simulink model "verify_DF_fixp16_alu"  (R2020b)
settings: Solver=FixedStepDiscrete  StartTime=0.0  StopTime=0.01  FixedStep=DSPBASampleTime  RelTol=1e-3  EnableMultiTasking=on
PreLoadFcn:
  | setup_verify_DF_fixp16_alu;
InitFcn:
  | setup_verify_DF_fixp16_alu;
values from neighbouring files (symbols this model uses):
  DSPBASampleTime = FoldingFactor / (ClockFrequency * 1e6)    (= 5e-06)    [setup_DF_fixp16_alu_av.m]    (also in setup_sim_DF_fixp16_alu.m; setup_verify_DF_fixp16_alu.m)
undefined symbols (not defined in the file or in its folder): I_max, Position_PI_Limit, sigbuilder_block
libraries: DSPBABase x7, foc_blocks x1
settings Model: Creator=bjeppese  LastModifiedBy=mhonman
settings DataIOCC: LimitDataPoints=on  SaveFormat=Array  ReturnWorkspaceOutputs=off
settings OptimizationCC: LifeSpan=inf
settings DebuggingCC: SolverPrmCheckMsg=warning  SFUnexpectedBacktrackingDiag=warning  SFNoUnconditionalDefaultTransitionDiag=warning  SFExecutionAtInitializationDiag=none  ArithmeticOperatorsInVariantConditions=warning
settings HardwareCC: ProdBitPerPointer=32  ProdBitPerSizeT=32  ProdBitPerPtrDiffT=32  ProdLargestAtomicFloat=None  ProdIntDivRoundTo=Undefined  ProdEndianess=Unspecified  ProdWordSize=32  ProdHWDeviceType=32-bit Generic
settings ModelReferenceCC: PropagateSignalLabelsOutOfModel=off
settings SFSimCC: SimUseLocalCustomCode=off  CustomCodeUndefinedFunction=UseInterfaceOnly
settings RTWCC: RTWUseLocalCustomCode=off
settings CodeAppCC: StateflowObjectComments=on
settings GRTTargetCC: TargetLangStandard=C89/C90 (ANSI)
settings ConfigComp: CovMetricSettings=dw  CovSaveCumulativeToWorkspaceVar=on  CovSaveSingleToWorkspaceVar=on  CovExternalEMLEnable=off

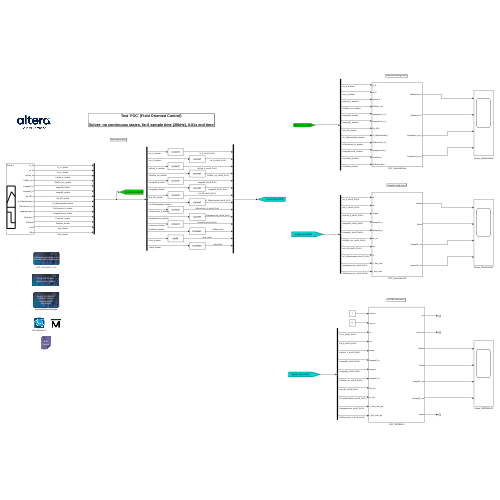
[thumbnail: Simulink's stored preview of the top-level diagram]
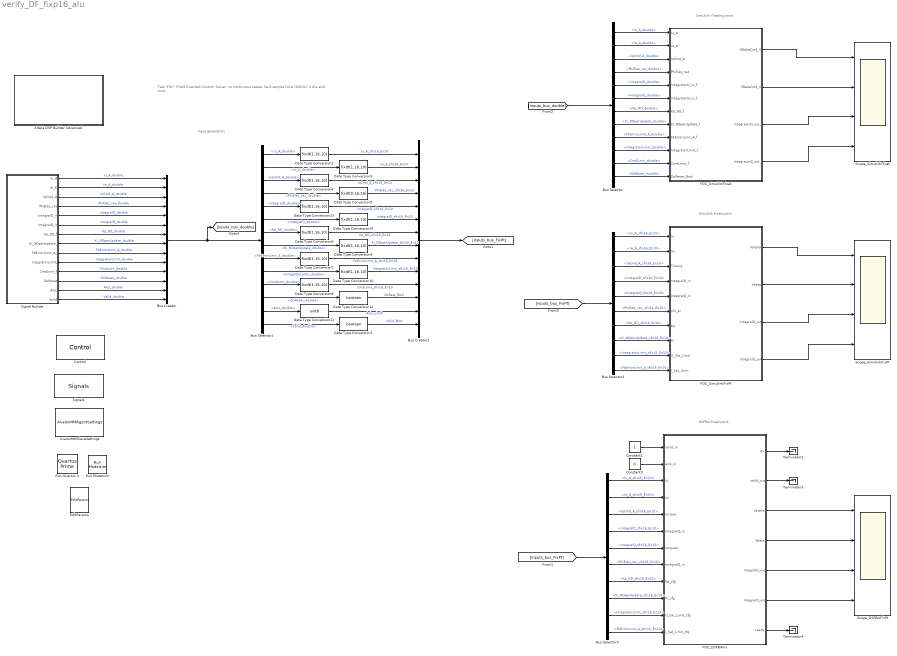
== system verify_DF_fixp16_alu ==
  note: Test 'FOC' (Field Oriented Control)
      |
      | Solver: no continuous states, 5e-6 sample time (20kHz), 0.01s end time
  note: DSPBA fixed point
  note: Input generation
  note: Simulink floating point
  note: Simulink fixed point
  Altera DSP Builder Advanced : Subsystem  mask(DSP Builder Advanced Blockset Ignored Block){}
      settings: OpenFcn=web('http://www.altera.com', '-new');
      mask Display: image(imread('alteralogo.tif'));
  AvalonMMSlaveSettings : DSPBABase/AvalonMMAgentSettings
  Bus Creator : BusCreator  Inputs=14
  Bus Creator1 : BusCreator  Inputs=14
  Bus Selector : BusSelector  OutputSignals=Iu_A_double,Iw_A_double,IqCmd_A_double,PhiElec_rev_double,IntegralD_double,IntegralQ_double,Kp_ND_double,Ki_NDperUpdate_double,FbErrorLimit_A_double,IntegratorLimit_double,CmdLimit_double,DoReset_double
  Bus Selector1 : BusSelector  OutputSignals=Iu_A_double,Iw_A_double,IqCmd_A_double,PhiElec_rev_double,IntegralD_double,IntegralQ_double,Kp_ND_double,Ki_NDperUpdate_double,FbErrorLimit_A_double,IntegratorLimit_double,CmdLimit_double,DoReset_double,Axis_double,Valid_double
  Bus Selector2 : BusSelector  OutputSignals=Iu_A_sfix16_En10,Iw_A_sfix16_En10,IqCmd_A_sfix16_En10,IntegralD_sfix16_En10,IntegralQ_sfix16_En10,PhiElec_rev_ufix16_En16,Kp_ND_sfix16_En10,Ki_NDperUpdate_sfix16_En10,IntegratorLimit_sfix16_En10,FbErrorLimit_A_sfix16_En10
  Bus Selector3 : BusSelector  OutputSignals=Iu_A_sfix16_En10,Iw_A_sfix16_En10,IqCmd_A_sfix16_En10,IntegralD_sfix16_En10,IntegralQ_sfix16_En10,PhiElec_rev_ufix16_En16,Kp_ND_sfix16_En10,Ki_NDperUpdate_sfix16_En10,IntegratorLimit_sfix16_En10,FbErrorLimit_A_sfix16_En10
  Constant1 : Constant  OutDataTypeStr=boolean
  Constant3 : Constant  Value=0  OutDataTypeStr=int32
  Control : DSPBABase/Control  generate=on  language=VHDL  destination=./rtlmax10  destination_gui=./rtlmax10  make_full_path=off  path_is_relative=on  autotestbench=on  signaldepth=2  coveragetestbench=off  logs=off  spacewidth=2  spacenum=1  addrwidth=6  datawidth=32  dataendian=Big Endian  hierarchicalnames=off  ramThresholdBits=-1  distRamThresholdBits=-1  mlabThresholdBits=-1  hardMultiplierThresholdLuts=-1  version=20090407  errorOnChanMismatch=1  errorOnGPIOMismatch=0  importModelsimResults=0  cycleAccurate=off  reinterpretCastMult=off  paramFile=overify_DF_fixp16_alu_params.xml
      settings: AttributesFormatString=HDL Generation is %<generate>
  Data Type Conversion1 : DataTypeConversion  OutDataTypeStr=boolean
  Data Type Conversion{2..4,6..10,13..14} (10 alike) : DataTypeConversion  OutDataTypeStr=fixdt(1,16,10)
  Data Type Conversion11 : DataTypeConversion  OutDataTypeStr=uint8
  Data Type Conversion12 : DataTypeConversion  OutDataTypeStr=boolean
  Data Type Conversion5 : DataTypeConversion  OutDataTypeStr=fixdt(0,16,16)
  EditParams : DSPBABase/EditParams  version=20090407
  FOC_DSPBAFix : Subsystem
  FOC_SimulinkFixPt : Subsystem
  FOC_SimulinkFloat : Subsystem
  Run Modelsim : DSPBABase/Run Modelsim  version=20090407
  Run Quartus II : DSPBABase/Quartus Prime  version=20090407
  Scope_DSPBAFixPt : Scope  NumInputPorts=4
  Scope_SimulinkFixPt : Scope  NumInputPorts=4
  Scope_SimulinkFloat : Scope  NumInputPorts=4
  Signal Builder : Subsystem  Tag=STV Subsys  LoadFcn=sigbuilder_block('load');  StartFcn=sigbuilder_block('start');  StopFcn=sigbuilder_block('stop');  ClipboardFcn=sigbuilder_block('clipboard');  mask(Sigbuilder block){tuvar=[0:10]}
      mask help: Simulink:masks:SigbuilderBlock_MD
      mask init:
      | if ~strcmp(get_param(bdroot(gcbh),'SimulationStatus'),'stopped') tuvar = sigbuilder_block('maskInit'); end
      settings: CopyFcn=sigbuilder_block('copy');  DeleteFcn=sigbuilder_block('delete');  ModelCloseFcn=sigbuilder_block('modelClose');  PreSaveFcn=sigbuilder_block('preSave');  PauseFcn=sigbuilder_block('pause');  ContinueFcn=sigbuilder_block('continue');  NameChangeFcn=sigbuilder_block('namechange');  OpenFcn=sigbuilder_block('open',[6 14.25 1428 732 ]);  CloseFcn=sigbuilder_block('close');
      mask Display: plot(0, 0, 100, 100,[2, 2, 32, 32, 2], [68, 8, 8, 68, 68],[32, 2], [38, 38], [32, 19, 2],[53, 60, 44], [32, 17, 17, 2],[16, 16, 31, 31]);txt = getActiveGroup(gcbh);text(2, 100, txt,'verticalAlignment', 'top');
  Signals : DSPBABase/Signals  clk=clk  freq=ClockFrequency  margin=0  rst=areset  rstactive=High  bus=bus  enbusclock=off  busfreq=100  bussync=on  version=20090407
  Terminator2 : Terminator
  Terminator3 : Terminator
  Terminator4 : Terminator
  wires:
  [inputs_bus_FixPt] -> Bus Selector3/1
  FOC_DSPBAFix/1(qv) -> Terminator2/1
  FOC_DSPBAFix/2(valid_out) -> Terminator3/1
  FOC_DSPBAFix/7(ready) -> Terminator4/1
  FOC_DSPBAFix/3(Valpha) -> Scope_DSPBAFixPt/1
  FOC_DSPBAFix/4(Vbeta) -> Scope_DSPBAFixPt/2
  Constant1/1 -> FOC_DSPBAFix/1(valid_in)
  Constant3/1 -> FOC_DSPBAFix/2(axis_in)
  Bus Selector3/1 -> FOC_DSPBAFix/3(Iu)  "<Iu_A_sfix16_En10>"
  Bus Selector3/2 -> FOC_DSPBAFix/4(Iw)  "<Iw_A_sfix16_En10>"
  Bus Selector3/3 -> FOC_DSPBAFix/5(torque)  "<IqCmd_A_sfix16_En10>"
  Bus Selector3/6 -> FOC_DSPBAFix/8(IntegralD_in)  "<PhiElec_rev_ufix16_En16>"
  Bus Selector3/7 -> FOC_DSPBAFix/9(Kp_cfg)  "<Kp_ND_sfix16_En10>"
  Bus Selector3/8 -> FOC_DSPBAFix/10(Ki_cfg)  "<Ki_NDperUpdate_sfix16_En10>"
  Bus Selector3/9 -> FOC_DSPBAFix/11(U_Sat_Limit_cfg)  "<IntegratorLimit_sfix16_En10>"
  Bus Selector3/10 -> FOC_DSPBAFix/12(I_Sat_Limit_cfg)  "<FbErrorLimit_A_sfix16_En10>"
  Bus Creator/1 -> [inputs_bus_double], Bus Selector1/1
  Bus Creator1/1 -> [inputs_bus_FixPt]
  Signal Builder/9(FbErrorLimit_A_f) -> Bus Creator/9  "FbErrorLimit_A_double"
  Signal Builder/7(Kp_ND_f) -> Bus Creator/7  "Kp_ND_double"
  Signal Builder/8(Ki_NDperUpdate_f) -> Bus Creator/8  "Ki_NDperUpdate_double"
  Signal Builder/10(IntegratorLimit_f) -> Bus Creator/10  "IntegratorLimit_double"
  Signal Builder/11(CmdLimit_f) -> Bus Creator/11  "CmdLimit_double"
  Signal Builder/12(DoReset) -> Bus Creator/12  "DoReset_double"
  Signal Builder/4(PhiElec_rev) -> Bus Creator/4  "PhiElec_rev_double"
  Signal Builder/3(IqCmd_A) -> Bus Creator/3  "IqCmd_A_double"
  Signal Builder/2(Iw_A) -> Bus Creator/2  "Iw_A_double"
  Bus Selector1/1 -> Data Type Conversion2/1  "<Iu_A_double>"
  Data Type Conversion2/1 -> Bus Creator1/1  "Iu_A_sfix16_En10"
  Bus Selector1/2 -> Data Type Conversion3/1  "<Iw_A_double>"
  Data Type Conversion3/1 -> Bus Creator1/2  "Iw_A_sfix16_En10"
  Bus Selector1/3 -> Data Type Conversion4/1  "<IqCmd_A_double>"
  Data Type Conversion4/1 -> Bus Creator1/3  "IqCmd_A_sfix16_En10"
  Bus Selector1/4 -> Data Type Conversion5/1  "<PhiElec_rev_double>"
  Data Type Conversion5/1 -> Bus Creator1/4  "PhiElec_rev_ufix16_En16"
  Bus Selector1/7 -> Data Type Conversion6/1  "<Kp_ND_double>"
  Data Type Conversion6/1 -> Bus Creator1/7  "Kp_ND_sfix16_En10"
  Bus Selector1/8 -> Data Type Conversion9/1  "<Ki_NDperUpdate_double>"
  Data Type Conversion9/1 -> Bus Creator1/8  "Ki_NDperUpdate_sfix16_En10"
  Bus Selector1/9 -> Data Type Conversion7/1  "<FbErrorLimit_A_double>"
  Data Type Conversion7/1 -> Bus Creator1/9  "FbErrorLimit_A_sfix16_En10"
  Bus Selector1/10 -> Data Type Conversion10/1  "<IntegratorLimit_double>"
  Data Type Conversion10/1 -> Bus Creator1/10  "IntegratorLimit_sfix16_En10"
  Bus Selector1/11 -> Data Type Conversion8/1  "<CmdLimit_double>"
  Data Type Conversion8/1 -> Bus Creator1/11  "CmdLimit_sfix16_En10"
  Bus Selector1/12 -> Data Type Conversion12/1  "<DoReset_double>"
  Signal Builder/13(Axis) -> Bus Creator/13  "Axis_double"
  Bus Selector1/13 -> Data Type Conversion11/1  "<Axis_double>"
  Data Type Conversion11/1 -> Bus Creator1/13  "Axis_uint8"
  Signal Builder/14(Valid) -> Bus Creator/14  "Valid_double"
  Data Type Conversion12/1 -> Bus Creator1/12  "DoRest_Bool"
  Bus Selector1/14 -> Data Type Conversion1/1  "<Valid_double>"
  Data Type Conversion1/1 -> Bus Creator1/14  "Valid_Bool"
  Signal Builder/1(Iu_A) -> Bus Creator/1  "Iu_A_double"
  Signal Builder/6(IntegralQ_in) -> Bus Creator/6  "IntegralQ_double"
  Signal Builder/5(IntegralD_in) -> Bus Creator/5  "IntegralD_double"
  Bus Selector1/5 -> Data Type Conversion13/1  "<IntegralD_double>"
  Data Type Conversion13/1 -> Bus Creator1/5  "IntegralD_sfix16_En10"
  Data Type Conversion14/1 -> Bus Creator1/6  "IntegralQ_sfix16_En10"
  Bus Selector1/6 -> Data Type Conversion14/1  "<IntegralQ_double>"
  Bus Selector3/4 -> FOC_DSPBAFix/6(IntegralQ_in)  "<IntegralD_sfix16_En10>"
  Bus Selector3/5 -> FOC_DSPBAFix/7(torque2)  "<IntegralQ_sfix16_En10>"
  FOC_DSPBAFix/5(IntegralD_out) -> Scope_DSPBAFixPt/3
  FOC_DSPBAFix/6(IntegralQ_out) -> Scope_DSPBAFixPt/4
  [inputs_bus_FixPt] -> Bus Selector2/1
  [inputs_bus_double] -> Bus Selector/1
  FOC_SimulinkFixPt/1(Valpha) -> Scope_SimulinkFixPt/1
  FOC_SimulinkFixPt/2(Vbeta) -> Scope_SimulinkFixPt/2
  FOC_SimulinkFloat/1(VAlphaCmd_V) -> Scope_SimulinkFloat/1
  FOC_SimulinkFloat/2(VBetaCmd_V) -> Scope_SimulinkFloat/2
  Bus Selector/1 -> FOC_SimulinkFloat/1(Iu_A)  "<Iu_A_double>"
  Bus Selector/2 -> FOC_SimulinkFloat/2(Iw_A)  "<Iw_A_double>"
  Bus Selector/3 -> FOC_SimulinkFloat/3(IqCmd_A)  "<IqCmd_A_double>"
  Bus Selector/4 -> FOC_SimulinkFloat/4(PhiElec_rad)  "<PhiElec_rev_double>"
  Bus Selector/7 -> FOC_SimulinkFloat/7(Kp_ND_f)  "<Kp_ND_double>"
  Bus Selector/8 -> FOC_SimulinkFloat/8(Ki_NDperUpdate_f)  "<Ki_NDperUpdate_double>"
  Bus Selector/9 -> FOC_SimulinkFloat/9(FbErrorLimit_A_f)  "<FbErrorLimit_A_double>"
  Bus Selector/10 -> FOC_SimulinkFloat/10(IntegratorLimit_f)  "<IntegratorLimit_double>"
  Bus Selector/11 -> FOC_SimulinkFloat/11(CmdLimit_f)  "<CmdLimit_double>"
  Bus Selector/12 -> FOC_SimulinkFloat/12(DoReset_Bool)  "<DoReset_double>"
  Bus Selector2/1 -> FOC_SimulinkFixPt/1(Iu)  "<Iu_A_sfix16_En10>"
  Bus Selector2/2 -> FOC_SimulinkFixPt/2(Iw)  "<Iw_A_sfix16_En10>"
  Bus Selector2/3 -> FOC_SimulinkFixPt/3(Torque)  "<IqCmd_A_sfix16_En10>"
  Bus Selector2/6 -> FOC_SimulinkFixPt/6(phi_el)  "<PhiElec_rev_ufix16_En16>"
  Bus Selector2/7 -> FOC_SimulinkFixPt/7(Kp)  "<Kp_ND_sfix16_En10>"
  Bus Selector2/8 -> FOC_SimulinkFixPt/8(Ki)  "<Ki_NDperUpdate_sfix16_En10>"
  Bus Selector2/9 -> FOC_SimulinkFixPt/9(U_Sat_Limit)  "<IntegratorLimit_sfix16_En10>"
  Bus Selector2/10 -> FOC_SimulinkFixPt/10(I_Sat_Limit)  "<FbErrorLimit_A_sfix16_En10>"
  Bus Selector2/4 -> FOC_SimulinkFixPt/4(IntegralD_in)  "<IntegralD_sfix16_En10>"
  Bus Selector2/5 -> FOC_SimulinkFixPt/5(IntegralQ_in)  "<IntegralQ_sfix16_En10>"
  FOC_SimulinkFixPt/3(IntegralD_out) -> Scope_SimulinkFixPt/3
  FOC_SimulinkFixPt/4(IntegralQ_out) -> Scope_SimulinkFixPt/4
  Bus Selector/5 -> FOC_SimulinkFloat/5(IntegratorD_in_f)  "<IntegralD_double>"
  Bus Selector/6 -> FOC_SimulinkFloat/6(IntegratorQ_in_f)  "<IntegralQ_double>"
  FOC_SimulinkFloat/3(IntegratorD_out_f) -> Scope_SimulinkFloat/3
  FOC_SimulinkFloat/4(IntegratorQ_out_f) -> Scope_SimulinkFloat/4

== system verify_DF_fixp16_alu/Altera DSP Builder Advanced ==

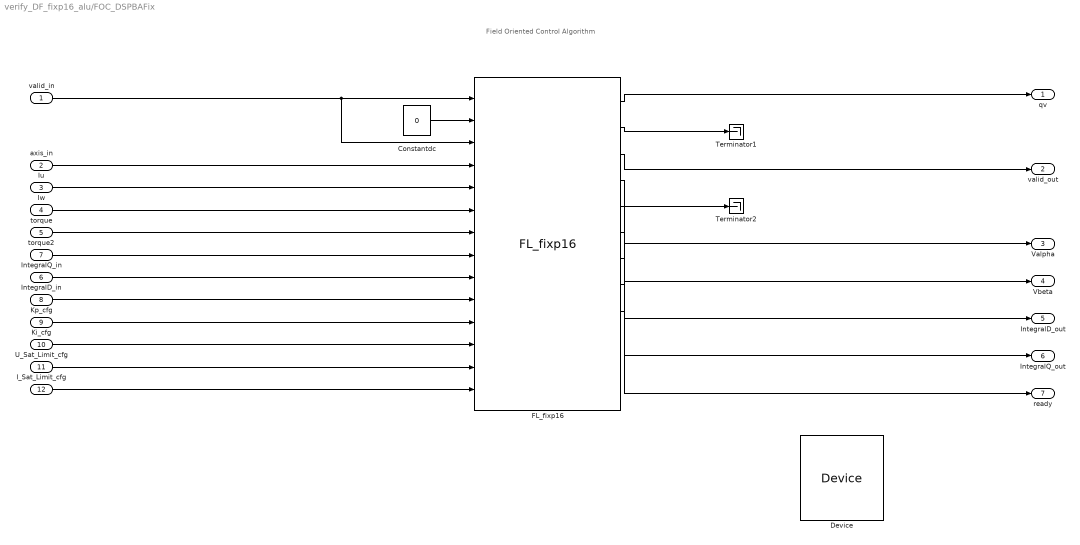
== system verify_DF_fixp16_alu/FOC_DSPBAFix ==
  note: Field Oriented Control Algorithm
  valid_in : Inport
  axis_in : Inport  Port=2
  Iu : Inport  Port=3
  Iw : Inport  Port=4
  torque : Inport  Port=5
  IntegralQ_in : Inport  Port=6
  torque2 : Inport  Port=7
  IntegralD_in : Inport  Port=8
  Kp_cfg : Inport  Port=9
  Ki_cfg : Inport  Port=10
  U_Sat_Limit_cfg : Inport  Port=11
  I_Sat_Limit_cfg : Inport  Port=12
  Constantdc : Constant  Value=0  OutDataTypeStr=uint8  SampleTime=DSPBASampleTime
  Device : DSPBABase/Device  family=MAX 10  deviceMember=Stratix V GX  stratix4device=Stratix IV E  hardcopy4device=HardCopy IV E  stratix5device=Stratix V GX  device=AUTO  speed=6  stratixSpeed=-5  stratix2Speed=-3  stratix3Speed=-2  stratix4gxSpeed=-2  stratix4gtSpeed=-1  cyclone2Speed=-6  cyclone3Speed=-7  arria2Speed=-4  cyclone4eSpeed=-8  stratix5Speed=-3  arria5Speed=-4  arriaSpeed=-6  cyclone3lsSpeed=-7  cyclone5Speed=-6  arria2gzSpeed=-3  nightFurySpeed=-2  ecp2Speed=-7  hardcopycompat=off  version=20140217  max10flashmode=off  max10nomeminit=off
  FL_fixp16 : foc_blocks/FL_fixp16  SystemSampleTime=-1  VariantActivationTime=update diagram  Latency=0  AutoFrameSizeCalculation=off
      link override ChannelOut1: latency=19
      settings: SourceProductName=FOC Blocks
  Terminator1 : Terminator
  Terminator2 : Terminator
  qv : Outport
  valid_out : Outport  Port=2
  Valpha : Outport  Port=3
  Vbeta : Outport  Port=4
  IntegralD_out : Outport  Port=5
  IntegralQ_out : Outport  Port=6
  ready : Outport  Port=7
  wires:
  FL_fixp16/5 -> Valpha/1
  FL_fixp16/1 -> qv/1
  FL_fixp16/3 -> valid_out/1
  FL_fixp16/6 -> Vbeta/1
  Constantdc/1 -> FL_fixp16/2
  FL_fixp16/8 -> IntegralQ_out/1
  FL_fixp16/7 -> IntegralD_out/1
  FL_fixp16/2 -> Terminator1/1
  valid_in/1 -> FL_fixp16/3, FL_fixp16/1
  Iu/1 -> FL_fixp16/5
  Iw/1 -> FL_fixp16/6
  torque/1 -> FL_fixp16/7
  IntegralD_in/1 -> FL_fixp16/10
  Kp_cfg/1 -> FL_fixp16/11
  Ki_cfg/1 -> FL_fixp16/12
  U_Sat_Limit_cfg/1 -> FL_fixp16/13
  axis_in/1 -> FL_fixp16/4
  FL_fixp16/9 -> ready/1
  FL_fixp16/4 -> Terminator2/1
  IntegralQ_in/1 -> FL_fixp16/9
  torque2/1 -> FL_fixp16/8
  I_Sat_Limit_cfg/1 -> FL_fixp16/14

== system verify_DF_fixp16_alu/FOC_SimulinkFixPt ==
  Iu : Inport
  Iw : Inport  Port=2
  Torque : Inport  Port=3
  IntegralD_in : Inport  Port=4
  IntegralQ_in : Inport  Port=5
  phi_el : Inport  Port=6
  Kp : Inport  Port=7
  Ki : Inport  Port=8
  U_Sat_Limit : Inport  Port=9
  I_Sat_Limit : Inport  Port=10
  FL_1 : Subsystem
  Valpha : Outport
  Vbeta : Outport  Port=2
  IntegralD_out : Outport  Port=3
  IntegralQ_out : Outport  Port=4
  wires:
  Iu/1 -> FL_1/1(Iu)
  Iw/1 -> FL_1/2(Iw)
  Torque/1 -> FL_1/3(Torque)
  phi_el/1 -> FL_1/6(phi_el)
  Kp/1 -> FL_1/7(Kp)
  Ki/1 -> FL_1/8(Ki)
  U_Sat_Limit/1 -> FL_1/9(U_Sat_Limit)
  I_Sat_Limit/1 -> FL_1/10(I_Sat_Limit)
  FL_1/1(Valpha) -> Valpha/1
  FL_1/2(Vbeta) -> Vbeta/1
  IntegralD_in/1 -> FL_1/5(IntegralD_in)
  IntegralQ_in/1 -> FL_1/4(IntegralQ_in)
  FL_1/3(IntegralD_out) -> IntegralD_out/1
  FL_1/4(IntegralQ_out) -> IntegralQ_out/1

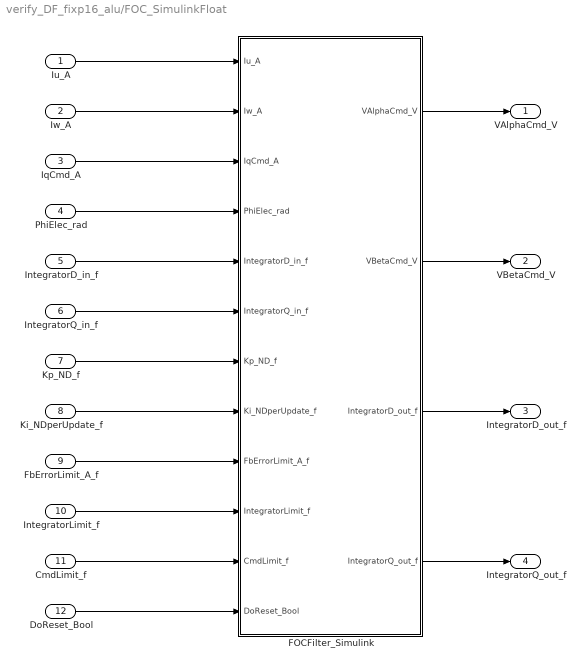
== system verify_DF_fixp16_alu/FOC_SimulinkFloat ==
  Iu_A : Inport
  Iw_A : Inport  Port=2
  IqCmd_A : Inport  Port=3
  PhiElec_rad : Inport  Port=4
  IntegratorD_in_f : Inport  Port=5
  IntegratorQ_in_f : Inport  Port=6
  Kp_ND_f : Inport  Port=7
  Ki_NDperUpdate_f : Inport  Port=8
  FbErrorLimit_A_f : Inport  Port=9
  IntegratorLimit_f : Inport  Port=10
  CmdLimit_f : Inport  Port=11
  DoReset_Bool : Inport  Port=12
  FOCFilter_Simulink : Subsystem
  VAlphaCmd_V : Outport
  VBetaCmd_V : Outport  Port=2
  IntegratorD_out_f : Outport  Port=3
  IntegratorQ_out_f : Outport  Port=4
  wires:
  IqCmd_A/1 -> FOCFilter_Simulink/3(IqCmd_A)
  Iu_A/1 -> FOCFilter_Simulink/1(Iu_A)
  Iw_A/1 -> FOCFilter_Simulink/2(Iw_A)
  PhiElec_rad/1 -> FOCFilter_Simulink/4(PhiElec_rad)
  Kp_ND_f/1 -> FOCFilter_Simulink/7(Kp_ND_f)
  Ki_NDperUpdate_f/1 -> FOCFilter_Simulink/8(Ki_NDperUpdate_f)
  FbErrorLimit_A_f/1 -> FOCFilter_Simulink/9(FbErrorLimit_A_f)
  IntegratorLimit_f/1 -> FOCFilter_Simulink/10(IntegratorLimit_f)
  CmdLimit_f/1 -> FOCFilter_Simulink/11(CmdLimit_f)
  DoReset_Bool/1 -> FOCFilter_Simulink/12(DoReset_Bool)
  FOCFilter_Simulink/1(VAlphaCmd_V) -> VAlphaCmd_V/1
  FOCFilter_Simulink/2(VBetaCmd_V) -> VBetaCmd_V/1
  IntegratorD_in_f/1 -> FOCFilter_Simulink/5(IntegratorD_in_f)
  IntegratorQ_in_f/1 -> FOCFilter_Simulink/6(IntegratorQ_in_f)
  FOCFilter_Simulink/3(IntegratorD_out_f) -> IntegratorD_out_f/1
  FOCFilter_Simulink/4(IntegratorQ_out_f) -> IntegratorQ_out_f/1

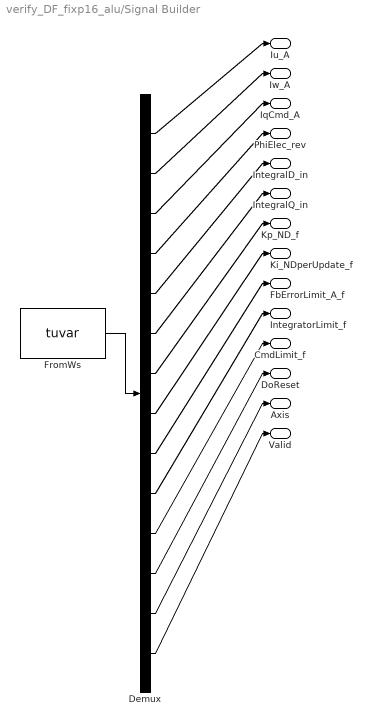
== system verify_DF_fixp16_alu/Signal Builder ==
  Demux : Demux  Tag=STV Demux  Outputs=14
      settings: DisplayOption=none
  FromWs : FromWorkspace  Tag=STV FromWs  VariableName=tuvar  SampleTime=DSPBASampleTime
      SigBuilderData=|
      | common.afterFinalStr = 'Extrapolate'
      | common.sampleTime = 'DSPBASampleTime'
      | dataSet.timeRange = [0 0.01]
      | dataSet.name = 'Group 1'
      | sbobj.Groups.Name = 'Group 1'
      | sbobj.Groups.Signals(1).Name = 'Iu_A'
      | sbobj.Groups.Signals(1).XData = [0 0.0011 0.0011 0.00256 0.00256 0.005 0.005 0.00625 0.00625 0.0075 0.0075 0.00875 0.00875 0.01]
      | sbobj.Groups.Signals(1).YData = [0 0 0.8 0.8 -0.6 -0.6 0.5 0.5 -0.6 -0.6 0.8 0.8 -0.85 -0.85]
      | sbobj.Groups.Signals(2).Name = 'Iw_A'
      | sbobj.Groups.Signals(2).XData = [0 0.00126 0.00126 0.00273 0.00273 0.00483 0.00483 0.00608 0.00608 0.0075 0.0075 0.00875 0.00875 0.01]
      | sbobj.Groups.Signals(2).YData = [0 0 0.7 0.7 -0.6 -0.6 0.6 0.6 -0.7 -0.7 0.6 0.6 -0.85 -0.85]
      | sbobj.Groups.Signals(3).Name = 'IqCmd_A'
      | sbobj.Groups.Signals(3).XData = [0 0.00146 0.00146 0.00292 0.00292 0.00473 0.00473 0.00595 0.00595 0.0075 0.0075 0.00875 0.00875 0.01]
      | sbobj.Groups.Signals(3).YData = [0 0 0.7 0.7 -0.95 -0.95 0.6 0.6 -0.8 -0.8 0.55 0.55 -0.7 -0.7]
      | sbobj.Groups.Signals(4).Name = 'PhiElec_rev'
      | sbobj.Groups.Signals(4).XData = [0 0.00161 0.00161 0.00309 0.00309 0.00462 0.00462 0.00582 0.00582 0.0075 0.0075 0.00875 0.00875 0.01]
      | sbobj.Groups.Signals(4).YData = [0 0 0.9 0.9 -0.95 -0.95 0.65 0.65 -0.95 -0.95 0.9 0.9 -0.65 -0.65]
      | sbobj.Groups.Signals(5).Name = 'IntegralD_in'
      | sbobj.Groups.Signals(5).XData = [0 0.00172 0.00172 0.0033 0.0033 0.00442 0.00442 0.00567 0.00567 0.0075 0.0075 0.00875 0.00875 0.01]
      | sbobj.Groups.Signals(5).YData = [0 0 0.65 0.65 -0.75 -0.75 0.8 0.8 -0.7 -0.7 0.8 0.8 -0.6 -0.6]
      | sbobj.Groups.Signals(6).Name = 'IntegralQ_in'
      | sbobj.Groups.Signals(6).XData = [0 0.00191 0.00191 0.00341 0.00341 0.00422 0.00422 0.00547 0.00547 0.0075 0.0075 0.00875 0.00875 0.01]
      | sbobj.Groups.Signals(6).YData = [0 0 0.8 0.8 -0.7 -0.7 0.8 0.8 -0.6 -0.6 0.7 0.7 -0.65 -0.65]
      | sbobj.Groups.Signals(7).Name = 'Kp_ND_f'
      | sbobj.Groups.Signals(7).XData = [0 0.01]
      | sbobj.Groups.Signals(7).YData = [0.1953125 0.1953125]
      | sbobj.Groups.Signals(8).Name = 'Ki_NDperUpdate_f'
      | sbobj.Groups.Signals(8).XData = [0 0.01]
      | sbobj.Groups.Signals(8).YData = [0.009765625 0.009765625]
      | sbobj.Groups.Signals(9).Name = 'FbErrorLimit_A_f'
      | sbobj.Groups.Signals(9).XData = [0 0.01]
      | sbobj.Groups.Signals(9).YData = [3.051757813 3.051757813]
      | sbobj.Groups.Signals(10).Name = 'IntegratorLimit_f'
      | sbobj.Groups.Signals(10).XData = [0 0.01]
      | sbobj.Groups.Signals(10).YData = [2.9296875 2.9296875]
      | sbobj.Groups.Signals(11).Name = 'CmdLimit_f'
      | sbobj.Groups.Signals(11).XData = [0 0.01]
      | sbobj.Groups.Signals(11).YData = [2.9296875 2.9296875]
      | sbobj.Groups.Signals(12).Name = 'DoReset'
      | sbobj.Groups.Signals(12).XData = [0 0.00047 0.00047 0.01]
      | sbobj.Groups.Signals(12).YData = [1 1 0 0]
      | sbobj.Groups.Signals(13).Name = 'Axis'
      | sbobj.Groups.Signals(13).XData = [0 0.01]
      | sbobj.Groups.Signals(13).YData = [0 0]
      | sbobj.Groups.Signals(14).Name = 'Valid'
      | sbobj.Groups.Signals(14).XData = [0 0.00066 0.00066 0.01]
      | sbobj.Groups.Signals(14).YData = [0 0 1 1]
      | sbobj.Groups.TimeRange = [0 0.01]
  Iu_A : Outport  Tag=STV Outport
  Iw_A : Outport  Tag=STV Outport  Port=2
  IqCmd_A : Outport  Tag=STV Outport  Port=3
  PhiElec_rev : Outport  Tag=STV Outport  Port=4
  IntegralD_in : Outport  Tag=STV Outport  Port=5
  IntegralQ_in : Outport  Tag=STV Outport  Port=6
  Kp_ND_f : Outport  Tag=STV Outport  Port=7
  Ki_NDperUpdate_f : Outport  Tag=STV Outport  Port=8
  FbErrorLimit_A_f : Outport  Tag=STV Outport  Port=9
  IntegratorLimit_f : Outport  Tag=STV Outport  Port=10
  CmdLimit_f : Outport  Tag=STV Outport  Port=11
  DoReset : Outport  Tag=STV Outport  Port=12
  Axis : Outport  Tag=STV Outport  Port=13
  Valid : Outport  Tag=STV Outport  Port=14
  wires:
  FromWs/1 -> Demux/1
  Demux/1 -> Iu_A/1
  Demux/2 -> Iw_A/1
  Demux/3 -> IqCmd_A/1
  Demux/4 -> PhiElec_rev/1
  Demux/5 -> IntegralD_in/1
  Demux/6 -> IntegralQ_in/1
  Demux/7 -> Kp_ND_f/1
  Demux/8 -> Ki_NDperUpdate_f/1
  Demux/9 -> FbErrorLimit_A_f/1
  Demux/10 -> IntegratorLimit_f/1
  Demux/11 -> CmdLimit_f/1
  Demux/12 -> DoReset/1
  Demux/13 -> Axis/1
  Demux/14 -> Valid/1

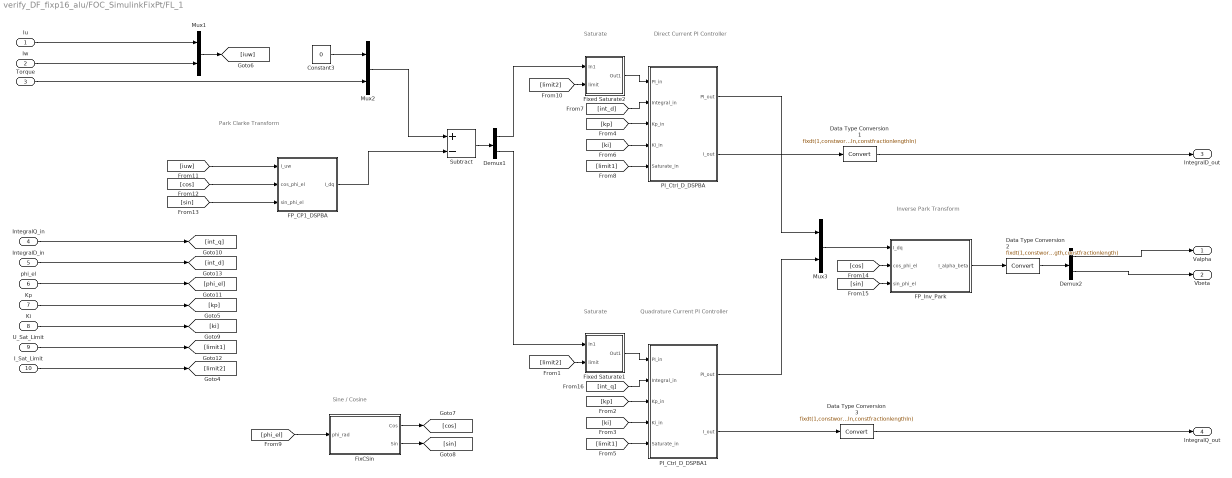
== system verify_DF_fixp16_alu/FOC_SimulinkFixPt/FL_1 ==
  note: Saturate
  note: Direct Current
      | PI Controller
  note: Saturate
  note: Quadrature Current
      | PI Controller
  note: Inverse Park
      |  Transform
  note: Park Clarke
      |  Transform
  note: Sine / Cosine
  Iu : Inport
  Iw : Inport  Port=2
  Torque : Inport  Port=3
  IntegralQ_in : Inport  Port=4
  IntegralD_in : Inport  Port=5
  phi_el : Inport  Port=6
  Kp : Inport  Port=7
  Ki : Inport  Port=8
  U_Sat_Limit : Inport  Port=9
  I_Sat_Limit : Inport  Port=10
  Constant3 : Constant  Value=0  OutDataTypeStr=fixdt(1,constwordlengthIn,constfractionlengthIn)
  Data Type Conversion1 : DataTypeConversion  OutDataTypeStr=fixdt(1,constwordlengthIn,constfractionlengthIn)
  Data Type Conversion2 : DataTypeConversion  OutDataTypeStr=fixdt(1,constwordlength,constfractionlength)
  Data Type Conversion3 : DataTypeConversion  OutDataTypeStr=fixdt(1,constwordlengthIn,constfractionlengthIn)
  Demux1 : Demux  Outputs=2
  Demux2 : Demux  Outputs=2
  FP_CP1_DSPBA : Subsystem  Description=Clarke & Park Transforms
      mask Display: color('white');port_label('output', 1, 'I_dq'); port_label('input', 1, 'I_uw');port_label('input', 2, 'cos_phi');port_label('input', 3, 'sin_phi');
  FP_Inv_Park : Subsystem  Description=Inverse Park & Clarke transforms
      mask Display: color('white');port_label('output', 1, 'V_alpha_beta'); port_label('input', 1, 'V_dq');port_label('input', 2, 'cos_phi');port_label('input', 3, 'sin_phi');
  FixCSin : Subsystem
      mask Display: color('white');fprintf('Fixed sin/cos(a)');port_label('input',1,'a');port_label('output',1,'Cos');port_label('output',2,'Sin');
  Fixed Saturate1 : Subsystem
  Fixed Saturate2 : Subsystem
  Mux1 : Mux  Inputs=2
  Mux2 : Mux  Inputs=2
  Mux3 : Mux  Inputs=2
  PI_Ctrl_D_DSPBA : Subsystem
  PI_Ctrl_D_DSPBA1 : Subsystem
  Subtract : Sum  Inputs=+-
  Valpha : Outport
  Vbeta : Outport  Port=2
  IntegralD_out : Outport  Port=3
  IntegralQ_out : Outport  Port=4
  wires:
  FP_Inv_Park/1(I_alpha_beta) -> Data Type Conversion2/1
  [limit2] -> Fixed Saturate2/2(limit)
  [ki] -> PI_Ctrl_D_DSPBA/4(Ki_in)
  Fixed Saturate2/1(Out1) -> PI_Ctrl_D_DSPBA/1(PI_in)
  [kp] -> PI_Ctrl_D_DSPBA/3(Kp_in)
  [limit1] -> PI_Ctrl_D_DSPBA/5(Saturate_in)
  PI_Ctrl_D_DSPBA/2(I_out) -> Data Type Conversion1/1
  Mux2/1 -> Subtract/1
  FP_CP1_DSPBA/1(I_dq) -> Subtract/2
  Iu/1 -> Mux1/1
  [sin] -> FP_CP1_DSPBA/3(sin_phi_el)
  Constant3/1 -> Mux2/1
  Kp/1 -> [kp]
  Data Type Conversion2/1 -> Demux2/1
  [cos] -> FP_CP1_DSPBA/2(cos_phi_el)
  Torque/1 -> Mux2/2
  [int_q] -> PI_Ctrl_D_DSPBA1/2(Integral_in)
  [iuw] -> FP_CP1_DSPBA/1(I_uw)
  Data Type Conversion1/1 -> IntegralD_out/1
  Mux1/1 -> [iuw]
  Iw/1 -> Mux1/2
  FixCSin/1(Cos) -> [cos]
  phi_el/1 -> [phi_el]
  IntegralQ_in/1 -> [int_q]
  Ki/1 -> [ki]
  [phi_el] -> FixCSin/1(phi_rad)
  IntegralD_in/1 -> [int_d]
  FixCSin/2(Sin) -> [sin]
  [limit2] -> Fixed Saturate1/2(limit)
  Fixed Saturate1/1(Out1) -> PI_Ctrl_D_DSPBA1/1(PI_in)
  [limit1] -> PI_Ctrl_D_DSPBA1/5(Saturate_in)
  [ki] -> PI_Ctrl_D_DSPBA1/4(Ki_in)
  [kp] -> PI_Ctrl_D_DSPBA1/3(Kp_in)
  Demux1/2 -> Fixed Saturate1/1(In1)
  PI_Ctrl_D_DSPBA1/2(I_out) -> Data Type Conversion3/1
  Subtract/1 -> Demux1/1
  PI_Ctrl_D_DSPBA/1(PI_out) -> Mux3/1
  Mux3/1 -> FP_Inv_Park/1(I_dq)
  [cos] -> FP_Inv_Park/2(cos_phi_el)
  Demux1/1 -> Fixed Saturate2/1(In1)
  PI_Ctrl_D_DSPBA1/1(PI_out) -> Mux3/2
  [int_d] -> PI_Ctrl_D_DSPBA/2(Integral_in)
  [sin] -> FP_Inv_Park/3(sin_phi_el)
  Demux2/1 -> Valpha/1
  Demux2/2 -> Vbeta/1
  Data Type Conversion3/1 -> IntegralQ_out/1
  I_Sat_Limit/1 -> [limit2]
  U_Sat_Limit/1 -> [limit1]

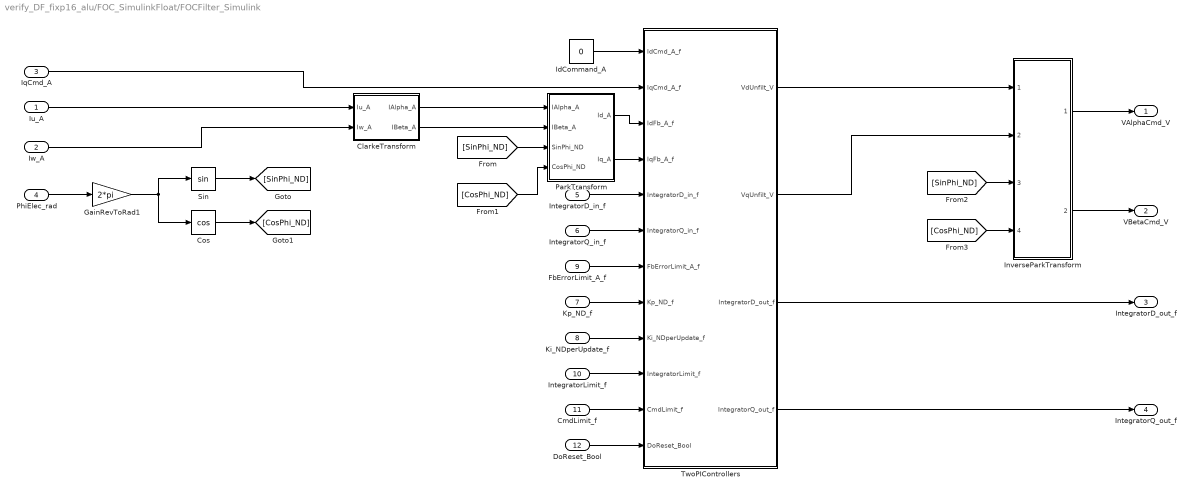
== system verify_DF_fixp16_alu/FOC_SimulinkFloat/FOCFilter_Simulink ==
  Iu_A : Inport
  Iw_A : Inport  Port=2
  IqCmd_A : Inport  Port=3
  PhiElec_rad : Inport  Port=4
  IntegratorD_in_f : Inport  Port=5
  IntegratorQ_in_f : Inport  Port=6
  Kp_ND_f : Inport  Port=7
  Ki_NDperUpdate_f : Inport  Port=8
  FbErrorLimit_A_f : Inport  Port=9
  IntegratorLimit_f : Inport  Port=10
  CmdLimit_f : Inport  Port=11
  DoReset_Bool : Inport  Port=12
  ClarkeTransform : Subsystem
  Cos : Trigonometry  Operator=cos
  GainRevToRad1 : Gain  Gain=2*pi
  IdCommand_A : Constant  Value=0
  InverseParkTransform : Subsystem
  ParkTransform : Subsystem
  Sin : Trigonometry
  TwoPIControllers : Subsystem
  VAlphaCmd_V : Outport
  VBetaCmd_V : Outport  Port=2
  IntegratorD_out_f : Outport  Port=3
  IntegratorQ_out_f : Outport  Port=4
  wires:
  InverseParkTransform/1(VAlphaCmd_V) -> VAlphaCmd_V/1
  FbErrorLimit_A_f/1 -> TwoPIControllers/7(FbErrorLimit_A_f)
  InverseParkTransform/2(VBetaCmd_V) -> VBetaCmd_V/1
  Kp_ND_f/1 -> TwoPIControllers/8(Kp_ND_f)
  Ki_NDperUpdate_f/1 -> TwoPIControllers/9(Ki_NDperUpdate_f)
  IntegratorLimit_f/1 -> TwoPIControllers/10(IntegratorLimit_f)
  CmdLimit_f/1 -> TwoPIControllers/11(CmdLimit_f)
  [CosPhi_ND] -> InverseParkTransform/4(CosPhi_ND)
  [SinPhi_ND] -> InverseParkTransform/3(SinPhi_ND)
  DoReset_Bool/1 -> TwoPIControllers/12(DoReset_Bool)
  TwoPIControllers/1(VdUnfilt_V) -> InverseParkTransform/1(VdCmd_V)
  Cos/1 -> [CosPhi_ND]
  Sin/1 -> [SinPhi_ND]
  TwoPIControllers/2(VqUnfilt_V) -> InverseParkTransform/2(VqCmd_V)
  [CosPhi_ND] -> ParkTransform/4(CosPhi_ND)
  [SinPhi_ND] -> ParkTransform/3(SinPhi_ND)
  ParkTransform/2(Iq_A) -> TwoPIControllers/4(IqFb_A_f)
  IdCommand_A/1 -> TwoPIControllers/1(IdCmd_A_f)
  ParkTransform/1(Id_A) -> TwoPIControllers/3(IdFb_A_f)
  PhiElec_rad/1 -> GainRevToRad1/1
  ClarkeTransform/1(IAlpha_A) -> ParkTransform/1(IAlpha_A)
  ClarkeTransform/2(IBeta_A) -> ParkTransform/2(IBeta_A)
  Iw_A/1 -> ClarkeTransform/2(Iw_A)
  Iu_A/1 -> ClarkeTransform/1(Iu_A)
  IqCmd_A/1 -> TwoPIControllers/2(IqCmd_A_f)
  GainRevToRad1/1 -> Sin/1, Cos/1
  IntegratorD_in_f/1 -> TwoPIControllers/5(IntegratorD_in_f)
  IntegratorQ_in_f/1 -> TwoPIControllers/6(IntegratorQ_in_f)
  TwoPIControllers/3(IntegratorD_out_f) -> IntegratorD_out_f/1
  TwoPIControllers/4(IntegratorQ_out_f) -> IntegratorQ_out_f/1

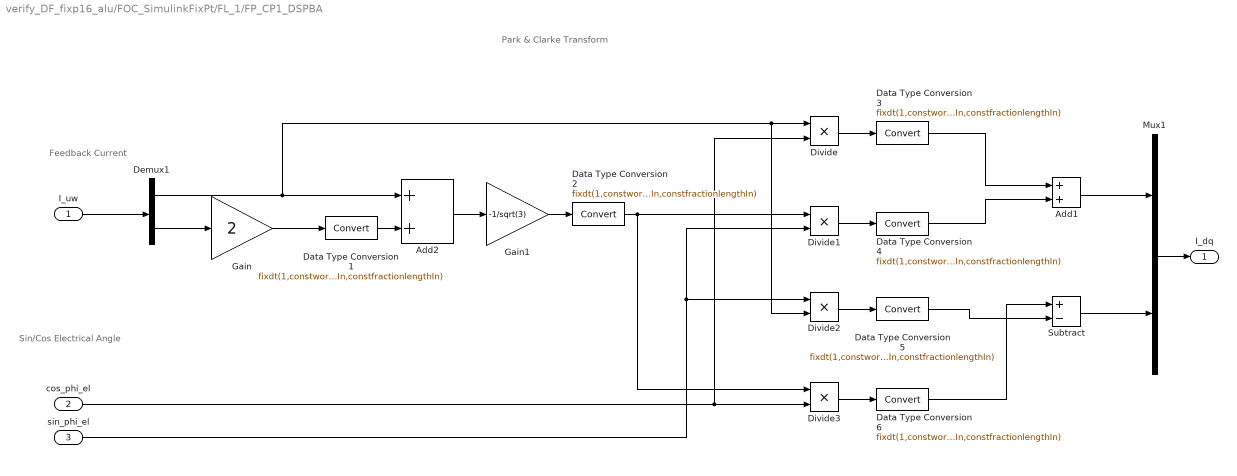
== system verify_DF_fixp16_alu/FOC_SimulinkFixPt/FL_1/FP_CP1_DSPBA ==
  note: Park & Clarke Transform
  note: Feedback Current
  note: Sin/Cos Electrical Angle
  I_uw : Inport
  cos_phi_el : Inport  Port=2
  sin_phi_el : Inport  Port=3
  Add1 : Sum
  Add2 : Sum
  Data Type Conversion{1..6} (6 alike) : DataTypeConversion  OutDataTypeStr=fixdt(1,constwordlengthIn,constfractionlengthIn)
  Demux1 : Demux  Outputs=2
  Divide{,1..3} (4 alike) : Product  Inputs=**  RndMeth=Zero  SaturateOnIntegerOverflow=on
  Gain : Gain  Gain=2
  Gain1 : Gain  Gain=-1/sqrt(3)
  Mux1 : Mux  Inputs=2
  Subtract : Sum  Inputs=+-
  I_dq : Outport
  wires:
  Subtract/1 -> Mux1/2
  Add1/1 -> Mux1/1
  Mux1/1 -> I_dq/1
  Data Type Conversion6/1 -> Subtract/1
  Data Type Conversion5/1 -> Subtract/2
  Data Type Conversion4/1 -> Add1/2
  Data Type Conversion3/1 -> Add1/1
  cos_phi_el/1 -> Divide/2, Divide3/2
  Data Type Conversion2/1 -> Divide3/1, Divide1/1
  Demux1/1 -> Divide2/2, Divide/1, Add2/1
  Demux1/2 -> Gain/1
  I_uw/1 -> Demux1/1
  sin_phi_el/1 -> Divide1/2, Divide2/1
  Data Type Conversion1/1 -> Add2/2
  Gain/1 -> Data Type Conversion1/1
  Add2/1 -> Gain1/1
  Gain1/1 -> Data Type Conversion2/1
  Divide/1 -> Data Type Conversion3/1
  Divide1/1 -> Data Type Conversion4/1
  Divide2/1 -> Data Type Conversion5/1
  Divide3/1 -> Data Type Conversion6/1

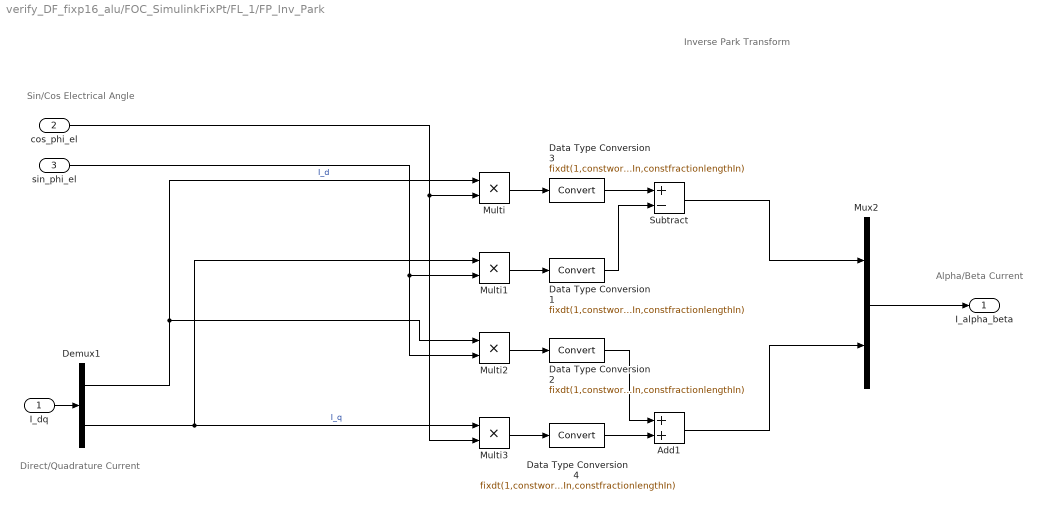
== system verify_DF_fixp16_alu/FOC_SimulinkFixPt/FL_1/FP_Inv_Park ==
  note: Inverse Park Transform
  note: Sin/Cos Electrical Angle
  note: Direct/Quadrature Current
  note: Alpha/Beta Current
  I_dq : Inport
  cos_phi_el : Inport  Port=2
  sin_phi_el : Inport  Port=3
  Add1 : Sum
  Data Type Conversion{1..4} (4 alike) : DataTypeConversion  OutDataTypeStr=fixdt(1,constwordlengthIn,constfractionlengthIn)
  Demux1 : Demux  Outputs=2
  Multi{,1..3} (4 alike) : Product  Inputs=**  RndMeth=Zero  SaturateOnIntegerOverflow=on
  Mux2 : Mux  Inputs=2
  Subtract : Sum  Inputs=+-
  I_alpha_beta : Outport
  wires:
  Data Type Conversion2/1 -> Add1/1
  Data Type Conversion4/1 -> Add1/2
  Data Type Conversion3/1 -> Subtract/1
  Data Type Conversion1/1 -> Subtract/2
  Demux1/1 -> Multi2/1, Multi/1  "I_d"
  cos_phi_el/1 -> Multi3/2, Multi/2
  Demux1/2 -> Multi3/1, Multi1/1  "I_q"
  sin_phi_el/1 -> Multi2/2, Multi1/2
  I_dq/1 -> Demux1/1
  Mux2/1 -> I_alpha_beta/1
  Subtract/1 -> Mux2/1
  Add1/1 -> Mux2/2
  Multi/1 -> Data Type Conversion3/1
  Multi1/1 -> Data Type Conversion1/1
  Multi2/1 -> Data Type Conversion2/1
  Multi3/1 -> Data Type Conversion4/1

== system verify_DF_fixp16_alu/FOC_SimulinkFixPt/FL_1/FixCSin ==
  note: Input format = uint(16)
      | covering range 0 to 2Pi Rad
  note: Fixed point Sin/Cos
  phi_rad : Inport
  Data Type Conversion1 : DataTypeConversion  OutDataTypeStr=fixdt(1,20,16)
  GainRevToRad1 : Gain  Gain=2*pi
  sincos : Trigonometry  Operator=sincos  ApproximationMethod=CORDIC  NumberOfIterations=19
  Cos : Outport
  Sin : Outport  Port=2
  wires:
  phi_rad/1 -> GainRevToRad1/1
  sincos/1 -> Sin/1
  Data Type Conversion1/1 -> sincos/1
  sincos/2 -> Cos/1
  GainRevToRad1/1 -> Data Type Conversion1/1

== system verify_DF_fixp16_alu/FOC_SimulinkFixPt/FL_1/Fixed Saturate1 ==
  In1 : Inport
  limit : Inport  Port=2
  CmpLT : RelationalOperator  Operator=<  OutDataTypeStr=boolean  RndMeth=Nearest
  CmpLT1 : RelationalOperator  OutDataTypeStr=boolean  RndMeth=Nearest
  Constant : Constant  Value=0  OutDataTypeStr=fixdt(1,constwordlengthIn,constfractionlengthIn)
  Subtract : Sum  Inputs=+-
  Switch : Switch  Criteria=u2 ~= 0  Threshold=Position_PI_Limit  ZeroCross=off
  Switch1 : Switch  Criteria=u2 ~= 0  Threshold=I_max  ZeroCross=off
  Out1 : Outport
  wires:
  Subtract/1 -> CmpLT/2, Switch1/1
  Switch1/1 -> Out1/1
  Switch/1 -> Switch1/3
  CmpLT/1 -> Switch1/2
  In1/1 -> CmpLT/1, Switch/3, CmpLT1/1
  limit/1 -> Subtract/2, CmpLT1/2, Switch/1
  Constant/1 -> Subtract/1
  CmpLT1/1 -> Switch/2

== system verify_DF_fixp16_alu/FOC_SimulinkFixPt/FL_1/Fixed Saturate2 ==
  In1 : Inport
  limit : Inport  Port=2
  CmpLT : RelationalOperator  Operator=<  OutDataTypeStr=boolean  RndMeth=Nearest
  CmpLT1 : RelationalOperator  OutDataTypeStr=boolean  RndMeth=Nearest
  Constant : Constant  Value=0  OutDataTypeStr=fixdt(1,constwordlengthIn,constfractionlengthIn)
  Subtract : Sum  Inputs=+-
  Switch : Switch  Criteria=u2 ~= 0  Threshold=Position_PI_Limit  ZeroCross=off
  Switch1 : Switch  Criteria=u2 ~= 0  Threshold=I_max  ZeroCross=off
  Out1 : Outport
  wires:
  CmpLT1/1 -> Switch/2
  Constant/1 -> Subtract/1
  limit/1 -> Switch/1, CmpLT1/2, Subtract/2
  In1/1 -> CmpLT1/1, Switch/3, CmpLT/1
  CmpLT/1 -> Switch1/2
  Switch/1 -> Switch1/3
  Switch1/1 -> Out1/1
  Subtract/1 -> Switch1/1, CmpLT/2

== system verify_DF_fixp16_alu/FOC_SimulinkFixPt/FL_1/PI_Ctrl_D_DSPBA ==
  note: Ki
  note: Kp
  note: Saturate Limit
  note: Integral Output
  note: Integral Input
  note: Correction Output
  note: Saturate
  note: Saturate
  note: Integral Gain
  note: Proportional Gain
  note: Error Input
  note: Simple Proportional + Integral (PI) Controller
  PI_in : Inport
  Integral_in : Inport  Port=2
  Kp_in : Inport  Port=3
  Ki_in : Inport  Port=4
  Saturate_in : Inport  Port=5
  Add : Sum
  Add1 : Sum
  Data Type Conversion1 : DataTypeConversion  OutDataTypeStr=fixdt(1,constwordlengthIn,constfractionlengthIn)
  Data Type Conversion3 : DataTypeConversion  OutDataTypeStr=fixdt(1,constwordlengthIn,constfractionlengthIn)
  Fixed Saturate1 : Subsystem
  Fixed Saturate2 : Subsystem
  Multi : Product  Inputs=**  RndMeth=Zero  SaturateOnIntegerOverflow=on
  Multi1 : Product  Inputs=**  RndMeth=Zero  SaturateOnIntegerOverflow=on
  PI_out : Outport
  I_out : Outport  Port=2
  wires:
  Multi1/1 -> Data Type Conversion1/1
  Multi/1 -> Data Type Conversion3/1
  Ki_in/1 -> Multi1/2
  Kp_in/1 -> Multi/2
  Saturate_in/1 -> Fixed Saturate2/2(limit), Fixed Saturate1/2(limit)
  Integral_in/1 -> Add/2
  Add/1 -> Fixed Saturate2/1(In1)
  Data Type Conversion1/1 -> Add/1
  Fixed Saturate2/1(Out1) -> Add1/2, I_out/1
  Data Type Conversion3/1 -> Add1/1
  PI_in/1 -> Multi/1, Multi1/1
  Add1/1 -> Fixed Saturate1/1(In1)
  Fixed Saturate1/1(Out1) -> PI_out/1

== system verify_DF_fixp16_alu/FOC_SimulinkFixPt/FL_1/PI_Ctrl_D_DSPBA1 ==
  note: Simple Proportional + Integral (PI) Controller
  note: Error Input
  note: Proportional Gain
  note: Integral Gain
  note: Saturate
  note: Saturate
  note: Correction Output
  note: Integral Input
  note: Integral Output
  note: Saturate Limit
  note: Kp
  note: Ki
  PI_in : Inport
  Integral_in : Inport  Port=2
  Kp_in : Inport  Port=3
  Ki_in : Inport  Port=4
  Saturate_in : Inport  Port=5
  Add : Sum
  Add1 : Sum
  Data Type Conversion1 : DataTypeConversion  OutDataTypeStr=fixdt(1,constwordlengthIn,constfractionlengthIn)
  Data Type Conversion3 : DataTypeConversion  OutDataTypeStr=fixdt(1,constwordlengthIn,constfractionlengthIn)
  Fixed Saturate1 : Subsystem
  Fixed Saturate2 : Subsystem
  Multi : Product  Inputs=**  RndMeth=Zero  SaturateOnIntegerOverflow=on
  Multi1 : Product  Inputs=**  RndMeth=Zero  SaturateOnIntegerOverflow=on
  PI_out : Outport
  I_out : Outport  Port=2
  wires:
  Fixed Saturate1/1(Out1) -> PI_out/1
  Add1/1 -> Fixed Saturate1/1(In1)
  PI_in/1 -> Multi1/1, Multi/1
  Data Type Conversion3/1 -> Add1/1
  Fixed Saturate2/1(Out1) -> I_out/1, Add1/2
  Data Type Conversion1/1 -> Add/1
  Add/1 -> Fixed Saturate2/1(In1)
  Integral_in/1 -> Add/2
  Saturate_in/1 -> Fixed Saturate1/2(limit), Fixed Saturate2/2(limit)
  Kp_in/1 -> Multi/2
  Ki_in/1 -> Multi1/2
  Multi/1 -> Data Type Conversion3/1
  Multi1/1 -> Data Type Conversion1/1

== system verify_DF_fixp16_alu/FOC_SimulinkFloat/FOCFilter_Simulink/ClarkeTransform ==
  note: IAlpha =  Iu
      | IBeta = -1/sqrt(3)*(Iu + 2*Iw)
  Iu_A : Inport
  Iw_A : Inport  Port=2
  Constant : Constant  Value=-1/sqrt(3)
  Divide : Product  Inputs=**
  Gain : Gain
  Gain1 : Gain  Gain=2
  Sum : Sum  Inputs=++|
  IAlpha_A : Outport
  IBeta_A : Outport  Port=2
  wires:
  Constant/1 -> Divide/2
  Gain/1 -> Sum/1, IAlpha_A/1  "IAlpha_A"
  Gain1/1 -> Sum/2
  Iw_A/1 -> Gain1/1
  Sum/1 -> Divide/1
  Iu_A/1 -> Gain/1
  Divide/1 -> IBeta_A/1

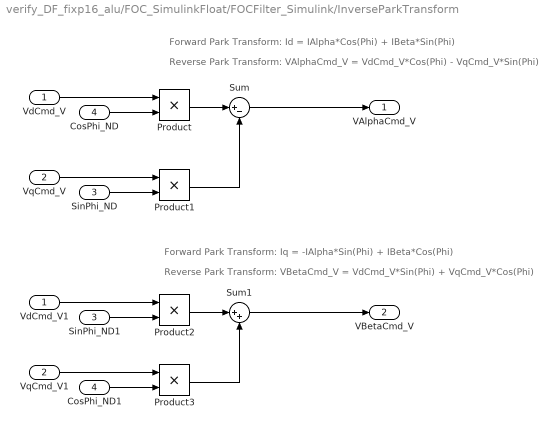
== system verify_DF_fixp16_alu/FOC_SimulinkFloat/FOCFilter_Simulink/InverseParkTransform ==
  note: Reverse Park Transform: VBetaCmd_V = VdCmd_V*Sin(Phi) + VqCmd_V*Cos(Phi)
  note: Reverse Park Transform: VAlphaCmd_V = VdCmd_V*Cos(Phi) - VqCmd_V*Sin(Phi)
  note: Forward Park Transform: Id = IAlpha*Cos(Phi) + IBeta*Sin(Phi)
  note: Forward Park Transform: Iq = -IAlpha*Sin(Phi) + IBeta*Cos(Phi)
  VdCmd_V : Inport
  VqCmd_V : Inport  Port=2
  SinPhi_ND : Inport  Port=3
  CosPhi_ND : Inport  Port=4
  CosPhi_ND1 : InportShadow  Port=4
  Product{,1..3} (4 alike) : Product
  SinPhi_ND1 : InportShadow  Port=3
  Sum : Sum  Inputs=|+-
  Sum1 : Sum  Inputs=|++
  VdCmd_V1 : InportShadow
  VqCmd_V1 : InportShadow  Port=2
  VAlphaCmd_V : Outport
  VBetaCmd_V : Outport  Port=2
  wires:
  VqCmd_V/1 -> Product1/1
  VdCmd_V/1 -> Product/1
  CosPhi_ND/1 -> Product/2
  SinPhi_ND/1 -> Product1/2
  Product/1 -> Sum/1
  Product1/1 -> Sum/2
  Sum/1 -> VAlphaCmd_V/1
  VdCmd_V1/1 -> Product2/1
  SinPhi_ND1/1 -> Product2/2
  VqCmd_V1/1 -> Product3/1
  CosPhi_ND1/1 -> Product3/2
  Product2/1 -> Sum1/1
  Product3/1 -> Sum1/2
  Sum1/1 -> VBetaCmd_V/1

== system verify_DF_fixp16_alu/FOC_SimulinkFloat/FOCFilter_Simulink/ParkTransform ==
  note: Iq = -IAlpha*Sin(Phi) + IBeta*Cos(Phi)
  note: Id = IAlpha*Cos(Phi) + IBeta*Sin(Phi)
  IAlpha_A : Inport
  IBeta_A : Inport  Port=2
  SinPhi_ND : Inport  Port=3
  CosPhi_ND : Inport  Port=4
  CosPhi_ND1 : InportShadow  Port=4
  IAlpha_A1 : InportShadow
  IBeta_A1 : InportShadow  Port=2
  Product{,1..3} (4 alike) : Product
  SinPhi_ND1 : InportShadow  Port=3
  Sum : Sum  Inputs=|++
  Sum1 : Sum  Inputs=|-+
  Id_A : Outport
  Iq_A : Outport  Port=2
  wires:
  Sum1/1 -> Iq_A/1
  Product3/1 -> Sum1/2
  Product2/1 -> Sum1/1
  CosPhi_ND1/1 -> Product3/2
  IBeta_A1/1 -> Product3/1
  SinPhi_ND1/1 -> Product2/2
  IAlpha_A1/1 -> Product2/1
  Sum/1 -> Id_A/1
  Product1/1 -> Sum/2
  Product/1 -> Sum/1
  SinPhi_ND/1 -> Product1/2
  CosPhi_ND/1 -> Product/2
  IAlpha_A/1 -> Product/1
  IBeta_A/1 -> Product1/1

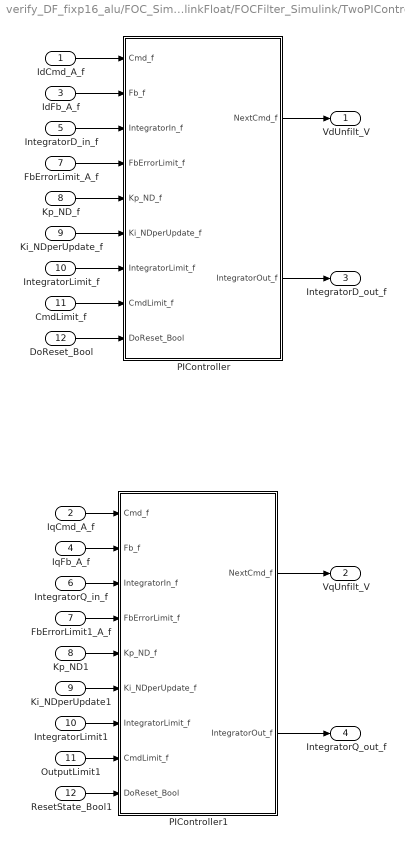
== system verify_DF_fixp16_alu/FOC_SimulinkFloat/FOCFilter_Simulink/TwoPIControllers ==
  IdCmd_A_f : Inport
  IqCmd_A_f : Inport  Port=2
  IdFb_A_f : Inport  Port=3
  IqFb_A_f : Inport  Port=4
  IntegratorD_in_f : Inport  Port=5
  IntegratorQ_in_f : Inport  Port=6
  FbErrorLimit_A_f : Inport  Port=7
  Kp_ND_f : Inport  Port=8
  Ki_NDperUpdate_f : Inport  Port=9
  IntegratorLimit_f : Inport  Port=10
  CmdLimit_f : Inport  Port=11
  DoReset_Bool : Inport  Port=12
  FbErrorLimit1_A_f : InportShadow  Port=7
  IntegratorLimit1 : InportShadow  Port=10
  Ki_NDperUpdate1 : InportShadow  Port=9
  Kp_ND1 : InportShadow  Port=8
  OutputLimit1 : InportShadow  Port=11
  PIController : Subsystem
  PIController1 : Subsystem
  ResetState_Bool1 : InportShadow  Port=12
  VdUnfilt_V : Outport
  VqUnfilt_V : Outport  Port=2
  IntegratorD_out_f : Outport  Port=3
  IntegratorQ_out_f : Outport  Port=4
  wires:
  FbErrorLimit_A_f/1 -> PIController/4(FbErrorLimit_f)
  Kp_ND_f/1 -> PIController/5(Kp_ND_f)
  Ki_NDperUpdate_f/1 -> PIController/6(Ki_NDperUpdate_f)
  IntegratorLimit_f/1 -> PIController/7(IntegratorLimit_f)
  CmdLimit_f/1 -> PIController/8(CmdLimit_f)
  DoReset_Bool/1 -> PIController/9(DoReset_Bool)
  IqCmd_A_f/1 -> PIController1/1(Cmd_f)
  IqFb_A_f/1 -> PIController1/2(Fb_f)
  FbErrorLimit1_A_f/1 -> PIController1/4(FbErrorLimit_f)
  Kp_ND1/1 -> PIController1/5(Kp_ND_f)
  Ki_NDperUpdate1/1 -> PIController1/6(Ki_NDperUpdate_f)
  IntegratorLimit1/1 -> PIController1/7(IntegratorLimit_f)
  OutputLimit1/1 -> PIController1/8(CmdLimit_f)
  ResetState_Bool1/1 -> PIController1/9(DoReset_Bool)
  PIController1/1(NextCmd_f) -> VqUnfilt_V/1
  IdFb_A_f/1 -> PIController/2(Fb_f)
  PIController/1(NextCmd_f) -> VdUnfilt_V/1
  IdCmd_A_f/1 -> PIController/1(Cmd_f)
  IntegratorD_in_f/1 -> PIController/3(IntegratorIn_f)
  IntegratorQ_in_f/1 -> PIController1/3(IntegratorIn_f)
  PIController/2(IntegratorOut_f) -> IntegratorD_out_f/1
  PIController1/2(IntegratorOut_f) -> IntegratorQ_out_f/1

== system verify_DF_fixp16_alu/FOC_SimulinkFixPt/FL_1/PI_Ctrl_D_DSPBA/Fixed Saturate1 ==
  In1 : Inport
  limit : Inport  Port=2
  CmpLT : RelationalOperator  Operator=<  OutDataTypeStr=boolean  RndMeth=Nearest
  CmpLT1 : RelationalOperator  OutDataTypeStr=boolean  RndMeth=Nearest
  Constant : Constant  Value=0  OutDataTypeStr=fixdt(1,constwordlengthIn,constfractionlengthIn)
  Subtract : Sum  Inputs=+-
  Switch : Switch  Criteria=u2 ~= 0  Threshold=Position_PI_Limit  ZeroCross=off
  Switch1 : Switch  Criteria=u2 ~= 0  Threshold=I_max  ZeroCross=off
  Out1 : Outport
  wires:
  Subtract/1 -> CmpLT/2, Switch1/1
  Switch1/1 -> Out1/1
  Switch/1 -> Switch1/3
  CmpLT/1 -> Switch1/2
  In1/1 -> CmpLT/1, Switch/3, CmpLT1/1
  limit/1 -> Subtract/2, CmpLT1/2, Switch/1
  Constant/1 -> Subtract/1
  CmpLT1/1 -> Switch/2

== system verify_DF_fixp16_alu/FOC_SimulinkFixPt/FL_1/PI_Ctrl_D_DSPBA/Fixed Saturate2 ==
  In1 : Inport
  limit : Inport  Port=2
  CmpLT : RelationalOperator  Operator=<  OutDataTypeStr=boolean  RndMeth=Nearest
  CmpLT1 : RelationalOperator  OutDataTypeStr=boolean  RndMeth=Nearest
  Constant : Constant  Value=0  OutDataTypeStr=fixdt(1,constwordlengthIn,constfractionlengthIn)
  Subtract : Sum  Inputs=+-
  Switch : Switch  Criteria=u2 ~= 0  Threshold=Position_PI_Limit  ZeroCross=off
  Switch1 : Switch  Criteria=u2 ~= 0  Threshold=I_max  ZeroCross=off
  Out1 : Outport
  wires:
  CmpLT1/1 -> Switch/2
  Constant/1 -> Subtract/1
  limit/1 -> Switch/1, CmpLT1/2, Subtract/2
  In1/1 -> CmpLT1/1, Switch/3, CmpLT/1
  CmpLT/1 -> Switch1/2
  Switch/1 -> Switch1/3
  Switch1/1 -> Out1/1
  Subtract/1 -> Switch1/1, CmpLT/2

== system verify_DF_fixp16_alu/FOC_SimulinkFixPt/FL_1/PI_Ctrl_D_DSPBA1/Fixed Saturate1 ==
  In1 : Inport
  limit : Inport  Port=2
  CmpLT : RelationalOperator  Operator=<  OutDataTypeStr=boolean  RndMeth=Nearest
  CmpLT1 : RelationalOperator  OutDataTypeStr=boolean  RndMeth=Nearest
  Constant : Constant  Value=0  OutDataTypeStr=fixdt(1,constwordlengthIn,constfractionlengthIn)
  Subtract : Sum  Inputs=+-
  Switch : Switch  Criteria=u2 ~= 0  Threshold=Position_PI_Limit  ZeroCross=off
  Switch1 : Switch  Criteria=u2 ~= 0  Threshold=I_max  ZeroCross=off
  Out1 : Outport
  wires:
  CmpLT1/1 -> Switch/2
  Constant/1 -> Subtract/1
  limit/1 -> Switch/1, CmpLT1/2, Subtract/2
  In1/1 -> CmpLT1/1, Switch/3, CmpLT/1
  CmpLT/1 -> Switch1/2
  Switch/1 -> Switch1/3
  Switch1/1 -> Out1/1
  Subtract/1 -> Switch1/1, CmpLT/2

== system verify_DF_fixp16_alu/FOC_SimulinkFixPt/FL_1/PI_Ctrl_D_DSPBA1/Fixed Saturate2 ==
  In1 : Inport
  limit : Inport  Port=2
  CmpLT : RelationalOperator  Operator=<  OutDataTypeStr=boolean  RndMeth=Nearest
  CmpLT1 : RelationalOperator  OutDataTypeStr=boolean  RndMeth=Nearest
  Constant : Constant  Value=0  OutDataTypeStr=fixdt(1,constwordlengthIn,constfractionlengthIn)
  Subtract : Sum  Inputs=+-
  Switch : Switch  Criteria=u2 ~= 0  Threshold=Position_PI_Limit  ZeroCross=off
  Switch1 : Switch  Criteria=u2 ~= 0  Threshold=I_max  ZeroCross=off
  Out1 : Outport
  wires:
  Subtract/1 -> CmpLT/2, Switch1/1
  Switch1/1 -> Out1/1
  Switch/1 -> Switch1/3
  CmpLT/1 -> Switch1/2
  In1/1 -> CmpLT/1, Switch/3, CmpLT1/1
  limit/1 -> Subtract/2, CmpLT1/2, Switch/1
  Constant/1 -> Subtract/1
  CmpLT1/1 -> Switch/2

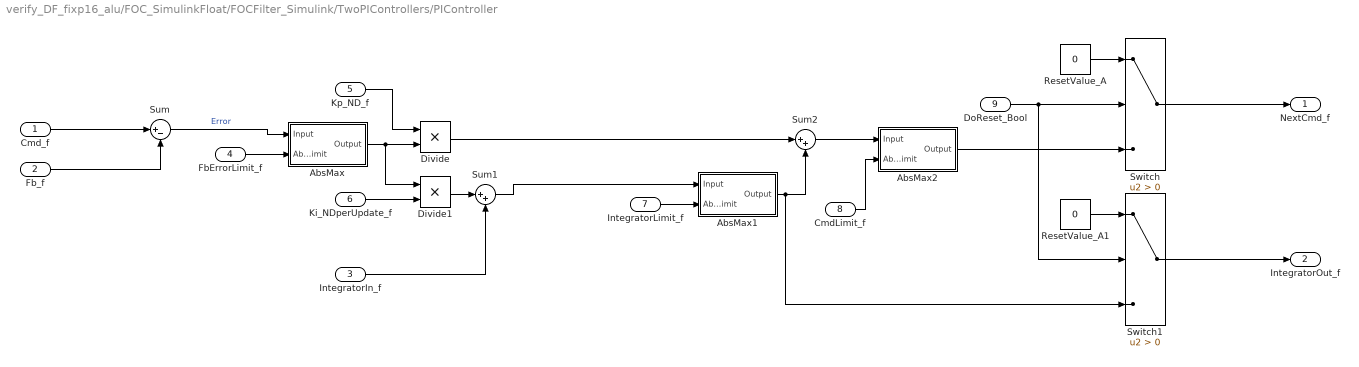
== system verify_DF_fixp16_alu/FOC_SimulinkFloat/FOCFilter_Simulink/TwoPIControllers/PIController ==
  Cmd_f : Inport
  Fb_f : Inport  Port=2
  IntegratorIn_f : Inport  Port=3
  FbErrorLimit_f : Inport  Port=4
  Kp_ND_f : Inport  Port=5
  Ki_NDperUpdate_f : Inport  Port=6
  IntegratorLimit_f : Inport  Port=7
  CmdLimit_f : Inport  Port=8
  DoReset_Bool : Inport  Port=9
  AbsMax : Subsystem
  AbsMax1 : Subsystem
  AbsMax2 : Subsystem
  Divide : Product  Inputs=**
  Divide1 : Product  Inputs=**
  ResetValue_A : Constant  Value=0
  ResetValue_A1 : Constant  Value=0
  Sum : Sum  Inputs=|+-
  Sum1 : Sum  Inputs=|++
  Sum2 : Sum  Inputs=|++
  Switch : Switch  Criteria=u2 > Threshold
  Switch1 : Switch  Criteria=u2 > Threshold
  NextCmd_f : Outport
  IntegratorOut_f : Outport  Port=2
  wires:
  IntegratorLimit_f/1 -> AbsMax1/2(AbsLimit)
  Switch1/1 -> IntegratorOut_f/1
  AbsMax2/1(Output) -> Switch/3
  DoReset_Bool/1 -> Switch/2, Switch1/2
  ResetValue_A/1 -> Switch/1
  Switch/1 -> NextCmd_f/1
  AbsMax1/1(Output) -> Sum2/2, Switch1/3
  Sum2/1 -> AbsMax2/1(Input)
  CmdLimit_f/1 -> AbsMax2/2(AbsLimit)
  ResetValue_A1/1 -> Switch1/1
  AbsMax/1(Output) -> Divide/2, Divide1/1
  Divide/1 -> Sum2/1
  Sum1/1 -> AbsMax1/1(Input)
  FbErrorLimit_f/1 -> AbsMax/2(AbsLimit)
  Kp_ND_f/1 -> Divide/1
  Divide1/1 -> Sum1/1
  Sum/1 -> AbsMax/1(Input)  "Error"
  Ki_NDperUpdate_f/1 -> Divide1/2
  Cmd_f/1 -> Sum/1
  Fb_f/1 -> Sum/2
  IntegratorIn_f/1 -> Sum1/2

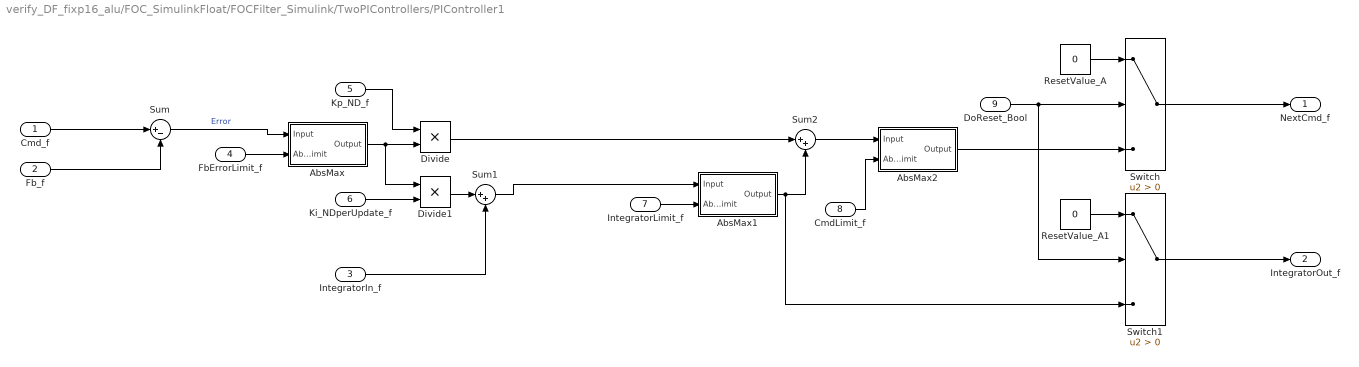
== system verify_DF_fixp16_alu/FOC_SimulinkFloat/FOCFilter_Simulink/TwoPIControllers/PIController1 ==
  Cmd_f : Inport
  Fb_f : Inport  Port=2
  IntegratorIn_f : Inport  Port=3
  FbErrorLimit_f : Inport  Port=4
  Kp_ND_f : Inport  Port=5
  Ki_NDperUpdate_f : Inport  Port=6
  IntegratorLimit_f : Inport  Port=7
  CmdLimit_f : Inport  Port=8
  DoReset_Bool : Inport  Port=9
  AbsMax : Subsystem
  AbsMax1 : Subsystem
  AbsMax2 : Subsystem
  Divide : Product  Inputs=**
  Divide1 : Product  Inputs=**
  ResetValue_A : Constant  Value=0
  ResetValue_A1 : Constant  Value=0
  Sum : Sum  Inputs=|+-
  Sum1 : Sum  Inputs=|++
  Sum2 : Sum  Inputs=|++
  Switch : Switch  Criteria=u2 > Threshold
  Switch1 : Switch  Criteria=u2 > Threshold
  NextCmd_f : Outport
  IntegratorOut_f : Outport  Port=2
  wires:
  IntegratorIn_f/1 -> Sum1/2
  Fb_f/1 -> Sum/2
  Cmd_f/1 -> Sum/1
  Ki_NDperUpdate_f/1 -> Divide1/2
  Sum/1 -> AbsMax/1(Input)  "Error"
  Divide1/1 -> Sum1/1
  Kp_ND_f/1 -> Divide/1
  FbErrorLimit_f/1 -> AbsMax/2(AbsLimit)
  Sum1/1 -> AbsMax1/1(Input)
  Divide/1 -> Sum2/1
  AbsMax/1(Output) -> Divide1/1, Divide/2
  ResetValue_A1/1 -> Switch1/1
  CmdLimit_f/1 -> AbsMax2/2(AbsLimit)
  Sum2/1 -> AbsMax2/1(Input)
  AbsMax1/1(Output) -> Switch1/3, Sum2/2
  Switch/1 -> NextCmd_f/1
  ResetValue_A/1 -> Switch/1
  DoReset_Bool/1 -> Switch1/2, Switch/2
  AbsMax2/1(Output) -> Switch/3
  Switch1/1 -> IntegratorOut_f/1
  IntegratorLimit_f/1 -> AbsMax1/2(AbsLimit)

== system verify_DF_fixp16_alu/FOC_SimulinkFloat/FOCFilter_Simulink/TwoPIControllers/PIController/AbsMax ==
  Input : Inport
  AbsLimit : Inport  Port=2
  Abs : Abs
  Divide : Product  Inputs=**
  Min : MinMax  Inputs=2
  Sign : Signum
  Output : Outport
  wires:
  Input/1 -> Abs/1, Sign/1
  Sign/1 -> Divide/2
  Min/1 -> Divide/1
  Divide/1 -> Output/1
  Abs/1 -> Min/1
  AbsLimit/1 -> Min/2

== system verify_DF_fixp16_alu/FOC_SimulinkFloat/FOCFilter_Simulink/TwoPIControllers/PIController/AbsMax1 ==
  Input : Inport
  AbsLimit : Inport  Port=2
  Abs : Abs
  Divide : Product  Inputs=**
  Min : MinMax  Inputs=2
  Sign : Signum
  Output : Outport
  wires:
  AbsLimit/1 -> Min/2
  Abs/1 -> Min/1
  Divide/1 -> Output/1
  Min/1 -> Divide/1
  Sign/1 -> Divide/2
  Input/1 -> Sign/1, Abs/1

== system verify_DF_fixp16_alu/FOC_SimulinkFloat/FOCFilter_Simulink/TwoPIControllers/PIController/AbsMax2 ==
  Input : Inport
  AbsLimit : Inport  Port=2
  Abs : Abs
  Divide : Product  Inputs=**
  Min : MinMax  Inputs=2
  Sign : Signum
  Output : Outport
  wires:
  Input/1 -> Abs/1, Sign/1
  Sign/1 -> Divide/2
  Min/1 -> Divide/1
  Divide/1 -> Output/1
  Abs/1 -> Min/1
  AbsLimit/1 -> Min/2

== system verify_DF_fixp16_alu/FOC_SimulinkFloat/FOCFilter_Simulink/TwoPIControllers/PIController1/AbsMax ==
  Input : Inport
  AbsLimit : Inport  Port=2
  Abs : Abs
  Divide : Product  Inputs=**
  Min : MinMax  Inputs=2
  Sign : Signum
  Output : Outport
  wires:
  AbsLimit/1 -> Min/2
  Abs/1 -> Min/1
  Divide/1 -> Output/1
  Min/1 -> Divide/1
  Sign/1 -> Divide/2
  Input/1 -> Sign/1, Abs/1

== system verify_DF_fixp16_alu/FOC_SimulinkFloat/FOCFilter_Simulink/TwoPIControllers/PIController1/AbsMax1 ==
  Input : Inport
  AbsLimit : Inport  Port=2
  Abs : Abs
  Divide : Product  Inputs=**
  Min : MinMax  Inputs=2
  Sign : Signum
  Output : Outport
  wires:
  Input/1 -> Abs/1, Sign/1
  Sign/1 -> Divide/2
  Min/1 -> Divide/1
  Divide/1 -> Output/1
  Abs/1 -> Min/1
  AbsLimit/1 -> Min/2

== system verify_DF_fixp16_alu/FOC_SimulinkFloat/FOCFilter_Simulink/TwoPIControllers/PIController1/AbsMax2 ==
  Input : Inport
  AbsLimit : Inport  Port=2
  Abs : Abs
  Divide : Product  Inputs=**
  Min : MinMax  Inputs=2
  Sign : Signum
  Output : Outport
  wires:
  AbsLimit/1 -> Min/2
  Abs/1 -> Min/1
  Divide/1 -> Output/1
  Min/1 -> Divide/1
  Sign/1 -> Divide/2
  Input/1 -> Sign/1, Abs/1
